simulink model "coneDetectorSim"  (R2023b)
settings: Solver=VariableStepAuto  StartTime=0.0  StopTime=33.26  RelTol=1e-3
undefined symbols (not defined in the file or in its folder): gray
libraries: dspvision x2, visiongeotforms x1
settings Model: Creator=hemant  LastModifiedBy=hemant
settings SolverCC: AlgebraicLoopSolver=TrustRegion
settings DebuggingCC: UnconnectedInputMsg=warning  UnconnectedOutputMsg=warning  UnconnectedLineMsg=warning
settings ModelReferenceCC: EnableRefExpFcnMdlSchedulingChecks=on
settings RTWCC: DLArmComputeVersion=19.05

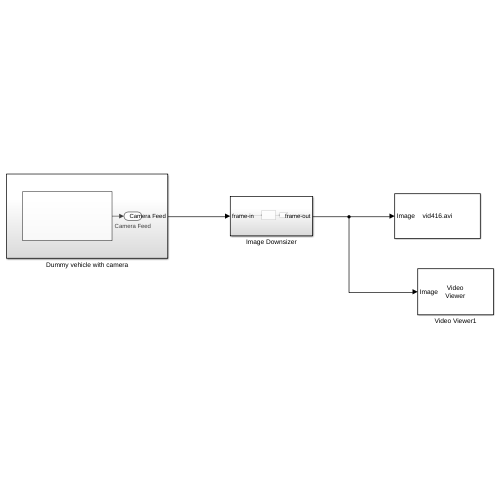
[thumbnail: Simulink's stored preview of the top-level diagram]
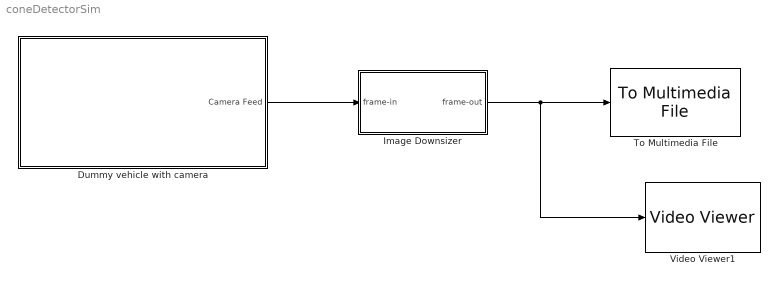
== system coneDetectorSim ==
  Dummy vehicle with camera : Subsystem
  Image Downsizer : Subsystem
  To Multimedia File : dspvision/To Multimedia File  outputFilename=vid416.avi  streamSelection=Video only  videoCompressor=MJPEG Compressor  audioCompressor=None (uncompressed)  imagePorts=One multidimensional signal  fileType=AVI  audioDatatype=Determine from input data type  fourcc=RGB  videoQuality=100  mj2000CompFactor=10
  Video Viewer1 : VideoViewer  colormapValue=gray(256)  FigPos=[827 610 426 411]
  wires:
  Dummy vehicle with camera/1(Camera Feed) -> Image Downsizer/1(frame-in)
  Image Downsizer/1(frame-out) -> Video Viewer1/1, To Multimedia File/1

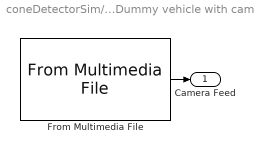
== system coneDetectorSim/Dummy vehicle with camera ==
  From Multimedia File : dspvision/From Multimedia File  inputFilename=/home/hemant/Projects/MATLAB/cone-detection-driverless-solution/camFeed.avi  readRange=[1 Inf]  loop=on  numPlays=inf  outputStreams=Video only  videoDataType=single  audioDataType=int16  inheritSampleTime=off  userDefinedSampleTime=1/50  noAudioOutput=off  isIntensityVideo=off  fourcc=RGB  colorVideoFormat=One multidimensional signal  outputEOF=off  dataOrg=Column-major  audioFrameSize=1024  computeAudioFrameSize=off  outSamplingMode=Sample based
  Camera Feed : Outport
  wires:
  From Multimedia File/1 -> Camera Feed/1

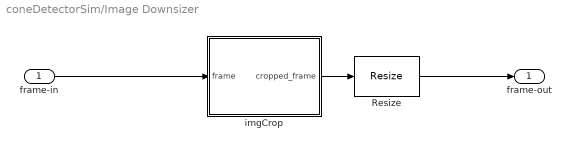
== system coneDetectorSim/Image Downsizer ==
  frame-in : Inport
  Resize : visiongeotforms/Resize  specify=Number of output rows and columns  rfactor=[200 150]  outCols=25  outRows=25  outRowsCols=[416 416]  interp_method=Bilinear  antialias=off  useROI=off  roiFlag=off  roundingMode=Nearest  overflowMode=on  prodOutputMode=Binary point scaling  prodOutputWordLength=32  prodOutputFracLength=10
  imgCrop : MATLAB Function  TreatAsAtomicUnit=on
  frame-out : Outport
  wires:
  imgCrop/1(cropped_frame) -> Resize/1
  frame-in/1 -> imgCrop/1(frame)
  Resize/1 -> frame-out/1

== matlab function coneDetectorSim/Image Downsizer/imgCrop ==
  data: frame input; cropped_frame output
function cropped_frame = fcn(frame)

cropped_frame = imcrop(frame, [281,1,719,719]);
